simulink model "case1"  (R2024b)
settings: Solver=FixedStepAuto  StartTime=0  StopTime=1  FixedStep=1e-7  RelTol=1e-3
values from neighbouring files (symbols this model uses):
  SG_D_1_D = 0.01056    [IEEE9_case_parameters.m]    (also in case1_parameters.m; case2_parameters.m; case3_parameters.m; case4_parameters.m)
  SG_D_1_EnableSaturation = 0    [IEEE9_case_parameters.m]    (also in case1_parameters.m; case2_parameters.m; case3_parameters.m; case4_parameters.m)
  SG_D_1_f0 = 60    [IEEE9_case_parameters.m]    (also in case1_parameters.m; case2_parameters.m; case3_parameters.m; case4_parameters.m)
  SG_D_1_H = 7.5    [IEEE9_case_parameters.m]    (also in case1_parameters.m; case2_parameters.m; case3_parameters.m; case4_parameters.m)
  SG_D_1_K_A = 20    [IEEE9_case_parameters.m]    (also in case1_parameters.m; case2_parameters.m; case3_parameters.m; case4_parameters.m)
  SG_D_1_K_E = 1.000000e+1    (= 10)    [IEEE9_case_parameters.m]    (also in case1_parameters.m; case2_parameters.m; case3_parameters.m; case4_parameters.m)
  SG_D_1_K_F = 2.363    [IEEE9_case_parameters.m]    (also in case1_parameters.m; case2_parameters.m; case3_parameters.m; case4_parameters.m)
  SG_D_1_K_s = 0.5    [IEEE9_case_parameters.m]    (also in case1_parameters.m = 5; case2_parameters.m = 5; case3_parameters.m = 5; case4_parameters.m = 5)
  SG_D_1_R_a = 0.001088    [IEEE9_case_parameters.m]    (also in case1_parameters.m; case2_parameters.m; case3_parameters.m; case4_parameters.m)
  SG_D_1_S_A = 1    [IEEE9_case_parameters.m]    (also in case1_parameters.m; case2_parameters.m; case3_parameters.m; case4_parameters.m)
  SG_D_1_S_B = 0.103    [IEEE9_case_parameters.m]    (also in case1_parameters.m; case2_parameters.m; case3_parameters.m; case4_parameters.m)
  SG_D_1_S_N = 10.659857    [IEEE9_case_parameters.m]    (also in case1_parameters.m; case2_parameters.m; case3_parameters.m; case4_parameters.m)
  SG_D_1_SpeedPara = 200    [IEEE9_case_parameters.m]    (also in case1_parameters.m; case2_parameters.m; case3_parameters.m; case4_parameters.m)
  SG_D_1_T_0 = 0.720173    [IEEE9_case_parameters.m]    (also in case1_parameters.m = 0.755522; case2_parameters.m = 0.808931; case3_parameters.m = 0.869402; case4_parameters.m = 0.729316)
  SG_D_1_T_1 = 0.3    [IEEE9_case_parameters.m]    (also in case1_parameters.m; case2_parameters.m; case3_parameters.m; case4_parameters.m)
  SG_D_1_T_2 = 0.05    [IEEE9_case_parameters.m]    (also in case1_parameters.m; case2_parameters.m; case3_parameters.m; case4_parameters.m)
  SG_D_1_T_3 = 0.02    [IEEE9_case_parameters.m]    (also in case1_parameters.m; case2_parameters.m; case3_parameters.m; case4_parameters.m)
  SG_D_1_T_4 = 0.005    [IEEE9_case_parameters.m]    (also in case1_parameters.m; case2_parameters.m; case3_parameters.m; case4_parameters.m)
  SG_D_1_T_A = 0.02    [IEEE9_case_parameters.m]    (also in case1_parameters.m; case2_parameters.m; case3_parameters.m; case4_parameters.m)
  SG_D_1_T_dd = 8.000000e+0    (= 8)    [IEEE9_case_parameters.m]    (also in case1_parameters.m; case2_parameters.m; case3_parameters.m; case4_parameters.m)
  SG_D_1_T_ddd = 0.04    [IEEE9_case_parameters.m]    (also in case1_parameters.m; case2_parameters.m; case3_parameters.m; case4_parameters.m)
  SG_D_1_T_E = 0.314    [IEEE9_case_parameters.m]    (also in case1_parameters.m; case2_parameters.m; case3_parameters.m; case4_parameters.m)
  SG_D_1_T_F = 0.35    [IEEE9_case_parameters.m]    (also in case1_parameters.m; case2_parameters.m; case3_parameters.m; case4_parameters.m)
  SG_D_1_T_qd = 0.8    [IEEE9_case_parameters.m]    (also in case1_parameters.m; case2_parameters.m; case3_parameters.m; case4_parameters.m)
  SG_D_1_T_qdd = 0.02    [IEEE9_case_parameters.m]    (also in case1_parameters.m; case2_parameters.m; case3_parameters.m; case4_parameters.m)
  SG_D_1_T_speed = 0.1    [IEEE9_case_parameters.m]    (also in case1_parameters.m = 200; case2_parameters.m = 200; case3_parameters.m = 200; case4_parameters.m = 200)
  SG_D_1_T_w = 0.5    [IEEE9_case_parameters.m]    (also in case1_parameters.m; case2_parameters.m; case3_parameters.m; case4_parameters.m)
  SG_D_1_V_ref = 1.990276    [IEEE9_case_parameters.m]    (also in case1_parameters.m = 2.042296; case2_parameters.m = 2.051388; case3_parameters.m = 2.089584; case4_parameters.m = 2.01845)
  SG_D_1_w_ref = 376.991118    [IEEE9_case_parameters.m]    (also in case1_parameters.m; case2_parameters.m; case3_parameters.m; case4_parameters.m)
  SG_D_1_wb = 6.000000e+1    (= 60)    [IEEE9_case_parameters.m]    (also in case1_parameters.m; case2_parameters.m; case3_parameters.m; case4_parameters.m)
  SG_D_1_x_d = 1.9    [IEEE9_case_parameters.m]    (also in case1_parameters.m; case2_parameters.m; case3_parameters.m; case4_parameters.m)
  SG_D_1_x_dd = 0.302    [IEEE9_case_parameters.m]    (also in case1_parameters.m; case2_parameters.m; case3_parameters.m; case4_parameters.m)
  SG_D_1_x_ddd = 0.204    [IEEE9_case_parameters.m]    (also in case1_parameters.m; case2_parameters.m; case3_parameters.m; case4_parameters.m)
  SG_D_1_x_l = 0.05    [IEEE9_case_parameters.m]    (also in case1_parameters.m; case2_parameters.m; case3_parameters.m; case4_parameters.m)
  SG_D_1_x_q = 1.3    [IEEE9_case_parameters.m]    (also in case1_parameters.m; case2_parameters.m; case3_parameters.m; case4_parameters.m)
  SG_D_1_x_qd = 0.5    [IEEE9_case_parameters.m]    (also in case1_parameters.m; case2_parameters.m; case3_parameters.m; case4_parameters.m)
  SG_D_1_x_qdd = 0.3    [IEEE9_case_parameters.m]    (also in case1_parameters.m; case2_parameters.m; case3_parameters.m; case4_parameters.m)
  SG_D_2_D = 0.02    [IEEE9_case_parameters.m]    (also in case1_parameters.m; case2_parameters.m; case3_parameters.m; case4_parameters.m)
  SG_D_2_EnableSaturation = 0    [IEEE9_case_parameters.m]    (also in case1_parameters.m; case2_parameters.m; case3_parameters.m; case4_parameters.m)
  SG_D_2_f0 = 60    [IEEE9_case_parameters.m]    (also in case1_parameters.m; case2_parameters.m; case3_parameters.m; case4_parameters.m)
  SG_D_2_H = 8.000000e+0    (= 8)    [IEEE9_case_parameters.m]    (also in case1_parameters.m; case2_parameters.m; case3_parameters.m; case4_parameters.m)
  SG_D_2_K_A = 20    [IEEE9_case_parameters.m]    (also in case1_parameters.m; case2_parameters.m; case3_parameters.m; case4_parameters.m)
  SG_D_2_K_E = 1.000000e+1    (= 10)    [IEEE9_case_parameters.m]    (also in case1_parameters.m; case2_parameters.m; case3_parameters.m; case4_parameters.m)
  SG_D_2_K_F = 2.363    [IEEE9_case_parameters.m]    (also in case1_parameters.m; case2_parameters.m; case3_parameters.m; case4_parameters.m)
  SG_D_2_K_s = 0.5    [IEEE9_case_parameters.m]    (also in case1_parameters.m = 4; case2_parameters.m = 4; case3_parameters.m = 4; case4_parameters.m = 4)
  SG_D_2_R_a = 0.001088    [IEEE9_case_parameters.m]    (also in case1_parameters.m; case2_parameters.m; case3_parameters.m; case4_parameters.m)
  SG_D_2_S_A = 1    [IEEE9_case_parameters.m]    (also in case1_parameters.m; case2_parameters.m; case3_parameters.m; case4_parameters.m)
  SG_D_2_S_B = 0.103    [IEEE9_case_parameters.m]    (also in case1_parameters.m; case2_parameters.m; case3_parameters.m; case4_parameters.m)
  SG_D_2_S_N = 10.659857    [IEEE9_case_parameters.m]    (also in case1_parameters.m; case2_parameters.m; case3_parameters.m; case4_parameters.m)
  SG_D_2_SpeedPara = 200    [IEEE9_case_parameters.m]    (also in case1_parameters.m; case2_parameters.m; case3_parameters.m; case4_parameters.m)
  SG_D_2_T_0 = 1.632913    [IEEE9_case_parameters.m]    (also in case1_parameters.m = 1.632925; case2_parameters.m = 1.632915; case3_parameters.m = 1.632914; case4_parameters.m = 1.632927)
  SG_D_2_T_1 = 0.2    [IEEE9_case_parameters.m]    (also in case1_parameters.m; case2_parameters.m; case3_parameters.m; case4_parameters.m)
  SG_D_2_T_2 = 0.05    [IEEE9_case_parameters.m]    (also in case1_parameters.m; case2_parameters.m; case3_parameters.m; case4_parameters.m)
  SG_D_2_T_3 = 0.02    [IEEE9_case_parameters.m]    (also in case1_parameters.m; case2_parameters.m; case3_parameters.m; case4_parameters.m)
  SG_D_2_T_4 = 0.005    [IEEE9_case_parameters.m]    (also in case1_parameters.m; case2_parameters.m; case3_parameters.m; case4_parameters.m)
  SG_D_2_T_A = 0.02    [IEEE9_case_parameters.m]    (also in case1_parameters.m; case2_parameters.m; case3_parameters.m; case4_parameters.m)
  SG_D_2_T_dd = 7.9    [IEEE9_case_parameters.m]    (also in case1_parameters.m; case2_parameters.m; case3_parameters.m; case4_parameters.m)
  SG_D_2_T_ddd = 0.04    [IEEE9_case_parameters.m]    (also in case1_parameters.m; case2_parameters.m; case3_parameters.m; case4_parameters.m)
  SG_D_2_T_E = 0.314    [IEEE9_case_parameters.m]    (also in case1_parameters.m; case2_parameters.m; case3_parameters.m; case4_parameters.m)
  SG_D_2_T_F = 0.35    [IEEE9_case_parameters.m]    (also in case1_parameters.m; case2_parameters.m; case3_parameters.m; case4_parameters.m)
  SG_D_2_T_qd = 0.8    [IEEE9_case_parameters.m]    (also in case1_parameters.m; case2_parameters.m; case3_parameters.m; case4_parameters.m)
  SG_D_2_T_qdd = 0.015    [IEEE9_case_parameters.m]    (also in case1_parameters.m; case2_parameters.m; case3_parameters.m; case4_parameters.m)
  SG_D_2_T_speed = 0.1    [IEEE9_case_parameters.m]    (also in case1_parameters.m = 150; case2_parameters.m = 150; case3_parameters.m = 150; case4_parameters.m = 150)
  SG_D_2_T_w = 0.35    [IEEE9_case_parameters.m]    (also in case1_parameters.m; case2_parameters.m; case3_parameters.m; case4_parameters.m)
  SG_D_2_V_ref = 2.58547    [IEEE9_case_parameters.m]    (also in case1_parameters.m = 2.597896; case2_parameters.m = 2.587136; case3_parameters.m = 2.586042; case4_parameters.m = 2.599679)
  SG_D_2_w_ref = 376.991118    [IEEE9_case_parameters.m]    (also in case1_parameters.m; case2_parameters.m; case3_parameters.m; case4_parameters.m)
  SG_D_2_wb = 6.000000e+1    (= 60)    [IEEE9_case_parameters.m]    (also in case1_parameters.m; case2_parameters.m; case3_parameters.m; case4_parameters.m)
  SG_D_2_x_d = 1.8    [IEEE9_case_parameters.m]    (also in case1_parameters.m; case2_parameters.m; case3_parameters.m; case4_parameters.m)
  SG_D_2_x_dd = 0.302    [IEEE9_case_parameters.m]    (also in case1_parameters.m; case2_parameters.m; case3_parameters.m; case4_parameters.m)
  SG_D_2_x_ddd = 0.204    [IEEE9_case_parameters.m]    (also in case1_parameters.m; case2_parameters.m; case3_parameters.m; case4_parameters.m)
  SG_D_2_x_l = 0.05    [IEEE9_case_parameters.m]    (also in case1_parameters.m; case2_parameters.m; case3_parameters.m; case4_parameters.m)
  SG_D_2_x_q = 1.25    [IEEE9_case_parameters.m]    (also in case1_parameters.m; case2_parameters.m; case3_parameters.m; case4_parameters.m)
  SG_D_2_x_qd = 0.5    [IEEE9_case_parameters.m]    (also in case1_parameters.m; case2_parameters.m; case3_parameters.m; case4_parameters.m)
  SG_D_2_x_qdd = 0.3    [IEEE9_case_parameters.m]    (also in case1_parameters.m; case2_parameters.m; case3_parameters.m; case4_parameters.m)
  SG_D_3_D = 0.02    [IEEE9_case_parameters.m]    (also in case1_parameters.m; case2_parameters.m; case3_parameters.m; case4_parameters.m)
  SG_D_3_EnableSaturation = 0    [IEEE9_case_parameters.m]    (also in case1_parameters.m; case2_parameters.m; case3_parameters.m; case4_parameters.m)
  SG_D_3_f0 = 60    [IEEE9_case_parameters.m]    (also in case1_parameters.m; case2_parameters.m; case3_parameters.m; case4_parameters.m)
  SG_D_3_H = 7.7    [IEEE9_case_parameters.m]    (also in case1_parameters.m; case2_parameters.m; case3_parameters.m; case4_parameters.m)
  SG_D_3_K_A = 20    [IEEE9_case_parameters.m]    (also in case1_parameters.m; case2_parameters.m; case3_parameters.m; case4_parameters.m)
  SG_D_3_K_E = 1.000000e+1    (= 10)    [IEEE9_case_parameters.m]    (also in case1_parameters.m; case2_parameters.m; case3_parameters.m; case4_parameters.m)
  SG_D_3_K_F = 2.363    [IEEE9_case_parameters.m]    (also in case1_parameters.m; case2_parameters.m; case3_parameters.m; case4_parameters.m)
  SG_D_3_K_s = 0.2    [IEEE9_case_parameters.m]    (also in case1_parameters.m = 2; case2_parameters.m = 2; case3_parameters.m = 2; case4_parameters.m = 2)
  SG_D_3_R_a = 0.001088    [IEEE9_case_parameters.m]    (also in case1_parameters.m; case2_parameters.m; case3_parameters.m; case4_parameters.m)
  SG_D_3_S_A = 1    [IEEE9_case_parameters.m]    (also in case1_parameters.m; case2_parameters.m; case3_parameters.m; case4_parameters.m)
  SG_D_3_S_B = 0.103    [IEEE9_case_parameters.m]    (also in case1_parameters.m; case2_parameters.m; case3_parameters.m; case4_parameters.m)
  SG_D_3_S_N = 10.659857    [IEEE9_case_parameters.m]    (also in case1_parameters.m; case2_parameters.m; case3_parameters.m; case4_parameters.m)
  SG_D_3_SpeedPara = 200    [IEEE9_case_parameters.m]    (also in case1_parameters.m; case2_parameters.m; case3_parameters.m; case4_parameters.m)
  SG_D_3_T_0 = 0.850788    [IEEE9_case_parameters.m]    (also in case1_parameters.m = 0.850786; case2_parameters.m = 0.850787; case3_parameters.m; case4_parameters.m = 0.850786)
  SG_D_3_T_1 = 0.2    [IEEE9_case_parameters.m]    (also in case1_parameters.m; case2_parameters.m; case3_parameters.m; case4_parameters.m)
  SG_D_3_T_2 = 0.05    [IEEE9_case_parameters.m]    (also in case1_parameters.m; case2_parameters.m; case3_parameters.m; case4_parameters.m)
  SG_D_3_T_3 = 0.02    [IEEE9_case_parameters.m]    (also in case1_parameters.m; case2_parameters.m; case3_parameters.m; case4_parameters.m)
  SG_D_3_T_4 = 0.005    [IEEE9_case_parameters.m]    (also in case1_parameters.m; case2_parameters.m; case3_parameters.m; case4_parameters.m)
  SG_D_3_T_A = 0.02    [IEEE9_case_parameters.m]    (also in case1_parameters.m; case2_parameters.m; case3_parameters.m; case4_parameters.m)
  SG_D_3_T_dd = 8.1    [IEEE9_case_parameters.m]    (also in case1_parameters.m; case2_parameters.m; case3_parameters.m; case4_parameters.m)
  SG_D_3_T_ddd = 0.04    [IEEE9_case_parameters.m]    (also in case1_parameters.m; case2_parameters.m; case3_parameters.m; case4_parameters.m)
  SG_D_3_T_E = 0.314    [IEEE9_case_parameters.m]    (also in case1_parameters.m; case2_parameters.m; case3_parameters.m; case4_parameters.m)
  SG_D_3_T_F = 0.35    [IEEE9_case_parameters.m]    (also in case1_parameters.m; case2_parameters.m; case3_parameters.m; case4_parameters.m)
  SG_D_3_T_qd = 0.8    [IEEE9_case_parameters.m]    (also in case1_parameters.m; case2_parameters.m; case3_parameters.m; case4_parameters.m)
  SG_D_3_T_qdd = 0.015    [IEEE9_case_parameters.m]    (also in case1_parameters.m; case2_parameters.m; case3_parameters.m; case4_parameters.m)
  SG_D_3_T_speed = 0.1    [IEEE9_case_parameters.m]    (also in case1_parameters.m = 180; case2_parameters.m = 180; case3_parameters.m = 180; case4_parameters.m = 180)
  SG_D_3_T_w = 0.4    [IEEE9_case_parameters.m]    (also in case1_parameters.m; case2_parameters.m; case3_parameters.m; case4_parameters.m)
  SG_D_3_V_ref = 1.892727    [IEEE9_case_parameters.m]    (also in case1_parameters.m = 1.906439; case2_parameters.m = 1.895535; case3_parameters.m = 1.892105; case4_parameters.m = 1.906598)
  SG_D_3_w_ref = 376.991118    [IEEE9_case_parameters.m]    (also in case1_parameters.m; case2_parameters.m; case3_parameters.m; case4_parameters.m)
  SG_D_3_wb = 6.000000e+1    (= 60)    [IEEE9_case_parameters.m]    (also in case1_parameters.m; case2_parameters.m; case3_parameters.m; case4_parameters.m)
  SG_D_3_x_d = 1.85    [IEEE9_case_parameters.m]    (also in case1_parameters.m; case2_parameters.m; case3_parameters.m; case4_parameters.m)
  SG_D_3_x_dd = 0.302    [IEEE9_case_parameters.m]    (also in case1_parameters.m; case2_parameters.m; case3_parameters.m; case4_parameters.m)
  SG_D_3_x_ddd = 0.204    [IEEE9_case_parameters.m]    (also in case1_parameters.m; case2_parameters.m; case3_parameters.m; case4_parameters.m)
  SG_D_3_x_l = 0.05    [IEEE9_case_parameters.m]    (also in case1_parameters.m; case2_parameters.m; case3_parameters.m; case4_parameters.m)
  SG_D_3_x_q = 1.2    [IEEE9_case_parameters.m]    (also in case1_parameters.m; case2_parameters.m; case3_parameters.m; case4_parameters.m)
  SG_D_3_x_qd = 0.5    [IEEE9_case_parameters.m]    (also in case1_parameters.m; case2_parameters.m; case3_parameters.m; case4_parameters.m)
  SG_D_3_x_qdd = 0.3    [IEEE9_case_parameters.m]    (also in case1_parameters.m; case2_parameters.m; case3_parameters.m; case4_parameters.m)
(part 7 of 12)

== system case1/SG_D_2/T_e_SG_D_2_block ==
  note: T_e_SG_D_2 in case1
      | $-\frac{\psi _{d,\mathrm{SG},D,2}\,\left(\psi _{q,\mathrm{SG},D,2}+\frac{\psi _{\mathrm{gq},\mathrm{SG},D,2}\,\left(x_{l}-x_{\mathrm{qdd}}\right)}{x_{l}-x_{\mathrm{qd}}}+\frac{\psi _{\mathrm{kq},\mathrm{SG},D,2}\,\left(x_{\mathrm{qd}}-x_{\mathrm{qdd}}\right)}{x_{l}-x_{\mathrm{qd}}}\right)}{x_{\mathrm{qdd}}}-\frac{\psi _{q,\mathrm{SG},D,2}\,\left(\frac{\psi _{\mathrm{1d},\mathrm{SG},D,2}\,\left(x_{\mathrm{dd}}-x_{\mathrm{ddd}}\right)}{x_{\mathrm{dd}}-x_{l}}-\psi _{d,\mathrm{SG},D,2}+\frac{\psi _{\mathrm{fd},\mathrm{SG},D,2}\,\left(x_{\mathrm{ddd}}-x_{l}\right)}{x_{\mathrm{dd}}-x_{l}}\right)}{x_{\mathrm{ddd}}}$
      | Automatically generated on 2025-10-31 18:49:09 .
  State_psi_d_SG_D_2_d17d7 : Inport
  State_psi_gq_SG_D_2_50ede : Inport  Port=2
  State_psi_kq_SG_D_2_ad282 : Inport  Port=3
  State_psi_q_SG_D_2_25b32 : Inport  Port=4
  State_psi_q_SG_D_2_fddea : Inport  Port=5
  State_psi_1d_SG_D_2_6821c : Inport  Port=6
  State_psi_d_SG_D_2_3bce2 : Inport  Port=7
  State_psi_fd_SG_D_2_27f6e : Inport  Port=8
  Add_23b6a : Sum
  Add_42760 : Sum
  Add_98a11 : Sum
  Add_aa7f3 : Sum
  Add_c8d0f : Sum
  Add_d49e1 : Sum
  Constant_-1_0fe01 : Constant  Value=-1
  Constant_-1_35857 : Constant  Value=-1
  Constant_-1_5d818 : Constant  Value=-1
  Constant_-1_78a66 : Constant  Value=-1
  Constant_-1_c3573 : Constant  Value=-1
  Constant_x_dd_09cbb : Constant  Value=x_dd
  Constant_x_dd_48c2b : Constant  Value=x_dd
  Constant_x_dd_a60eb : Constant  Value=x_dd
  Constant_x_ddd_2410b : Constant  Value=x_ddd
  Constant_x_ddd_26014 : Constant  Value=x_ddd
  Constant_x_ddd_6425f : Constant  Value=x_ddd
  Constant_x_l_05096 : Constant  Value=x_l
  Constant_x_l_3e3b1 : Constant  Value=x_l
  Constant_x_l_8c6a1 : Constant  Value=x_l
  Constant_x_l_93e72 : Constant  Value=x_l
  Constant_x_l_aba57 : Constant  Value=x_l
  Constant_x_l_c3be9 : Constant  Value=x_l
  Constant_x_qd_320b4 : Constant  Value=x_qd
  Constant_x_qd_56ce7 : Constant  Value=x_qd
  Constant_x_qd_8b2ca : Constant  Value=x_qd
  Constant_x_qdd_735f7 : Constant  Value=x_qdd
  Constant_x_qdd_e2b73 : Constant  Value=x_qdd
  Constant_x_qdd_e8dda : Constant  Value=x_qdd
  Divide_3759f : Product  Inputs=*/
  Divide_3be13 : Product  Inputs=*/
  Divide_9f252 : Product  Inputs=*/
  Divide_a3918 : Product  Inputs=*/
  Divide_aa95e : Product  Inputs=*/
  Divide_b0829 : Product  Inputs=*/
  Product_024a1 : Product
  Product_03878 : Product
  Product_2d239 : Product
  Product_3b454 : Product
  Product_4d8bd : Product
  Product_50cc2 : Product
  Product_5812c : Product
  Product_63870 : Product
  Product_da8e1 : Product
  Product_df83d : Product
  Product_e3721 : Product
  Subtract_283ed : Sum  Inputs=+-
  Subtract_3343d : Sum  Inputs=+-
  Subtract_51917 : Sum  Inputs=+-
  Subtract_708f3 : Sum  Inputs=+-
  Subtract_77632 : Sum  Inputs=+-
  Subtract_c6d03 : Sum  Inputs=+-
  Subtract_eb7e9 : Sum  Inputs=+-
  Blockout_T_e_SG_D_2_b65d9 : Outport
  wires:
  Constant_-1_5d818/1 -> Product_df83d/1
  Divide_a3918/1 -> Subtract_eb7e9/1
  Constant_-1_35857/1 -> Product_50cc2/1
  Constant_x_l_8c6a1/1 -> Product_50cc2/2
  Constant_x_qd_320b4/1 -> Subtract_51917/1
  Product_024a1/1 -> Divide_a3918/1
  Product_50cc2/1 -> Add_c8d0f/1
  Divide_aa95e/1 -> Subtract_3343d/2
  Constant_x_qdd_735f7/1 -> Subtract_51917/2
  Constant_x_qdd_e8dda/1 -> Divide_b0829/2
  Constant_x_ddd_6425f/1 -> Subtract_77632/2
  Constant_x_qdd_e2b73/1 -> Add_c8d0f/2
  Constant_x_l_93e72/1 -> Product_df83d/2
  Constant_-1_0fe01/1 -> Product_e3721/1
  Constant_x_l_3e3b1/1 -> Product_e3721/2
  Constant_-1_78a66/1 -> Product_03878/1
  State_psi_1d_SG_D_2_6821c/1 -> Product_03878/2
  Constant_x_dd_09cbb/1 -> Subtract_77632/1
  Divide_3be13/1 -> Subtract_eb7e9/2
  State_psi_gq_SG_D_2_50ede/1 -> Product_024a1/1
  Add_c8d0f/1 -> Product_024a1/2
  Subtract_eb7e9/1 -> Add_d49e1/1
  Constant_x_dd_48c2b/1 -> Subtract_708f3/1
  Product_df83d/1 -> Add_98a11/1
  Product_4d8bd/1 -> Product_5812c/1
  Constant_x_qd_56ce7/1 -> Add_98a11/2
  State_psi_kq_SG_D_2_ad282/1 -> Product_da8e1/1
  Subtract_51917/1 -> Product_da8e1/2
  Product_e3721/1 -> Add_aa7f3/1
  State_psi_q_SG_D_2_fddea/1 -> Product_63870/1
  Constant_x_qd_8b2ca/1 -> Add_aa7f3/2
  Product_03878/1 -> Product_2d239/1
  Divide_3759f/1 -> Add_23b6a/2
  Subtract_77632/1 -> Product_2d239/2
  Constant_x_l_c3be9/1 -> Subtract_708f3/2
  Constant_x_ddd_26014/1 -> Subtract_c6d03/1
  Constant_x_dd_a60eb/1 -> Subtract_283ed/1
  Constant_x_l_05096/1 -> Subtract_c6d03/2
  Add_23b6a/1 -> Blockout_T_e_SG_D_2_b65d9/1
  Add_98a11/1 -> Divide_a3918/2
  Product_da8e1/1 -> Divide_3be13/1
  Product_5812c/1 -> Divide_b0829/1
  State_psi_d_SG_D_2_d17d7/1 -> Product_4d8bd/2
  Add_aa7f3/1 -> Divide_3be13/2
  Product_2d239/1 -> Divide_9f252/1
  Subtract_708f3/1 -> Divide_9f252/2
  Constant_x_l_aba57/1 -> Subtract_283ed/2
  State_psi_fd_SG_D_2_27f6e/1 -> Product_3b454/1
  Constant_x_ddd_2410b/1 -> Divide_3759f/2
  Product_63870/1 -> Divide_3759f/1
  Subtract_c6d03/1 -> Product_3b454/2
  Divide_9f252/1 -> Add_42760/1
  State_psi_d_SG_D_2_3bce2/1 -> Add_42760/2
  Add_42760/1 -> Subtract_3343d/1
  Product_3b454/1 -> Divide_aa95e/1
  Subtract_283ed/1 -> Divide_aa95e/2
  Constant_-1_c3573/1 -> Product_4d8bd/1
  State_psi_q_SG_D_2_25b32/1 -> Add_d49e1/2
  Add_d49e1/1 -> Product_5812c/2
  Subtract_3343d/1 -> Product_63870/2
  Divide_b0829/1 -> Add_23b6a/1

== system case1/SG_D_2/d_E_fd_SG_D_2_block ==
  note: d_E_fd_SG_D_2 in case1
      | $\frac{V_{f,\mathrm{SG},D,2}-E_{\mathrm{fd},\mathrm{SG},D,2}\,K_{E}}{T_{E}}$
      | Automatically generated on 2025-10-31 18:48:51 .
  State_E_fd_SG_D_2_f3b44 : Inport
  State_V_f_SG_D_2_853e9 : Inport  Port=2
  Add_3a545 : Sum
  Constant_-1_cf921 : Constant  Value=-1
  Constant_K_E_ca9b5 : Constant  Value=K_E
  Constant_T_E_8d026 : Constant  Value=T_E
  Divide_8de38 : Product  Inputs=*/
  Product_ab2ba : Product
  Product_fb98c : Product
  Blockout_d_E_fd_SG_D_2_6e556 : Outport
  wires:
  Constant_-1_cf921/1 -> Product_fb98c/1
  State_E_fd_SG_D_2_f3b44/1 -> Product_fb98c/2
  Product_fb98c/1 -> Product_ab2ba/1
  Constant_K_E_ca9b5/1 -> Product_ab2ba/2
  Product_ab2ba/1 -> Add_3a545/1
  Constant_T_E_8d026/1 -> Divide_8de38/2
  State_V_f_SG_D_2_853e9/1 -> Add_3a545/2
  Add_3a545/1 -> Divide_8de38/1
  Divide_8de38/1 -> Blockout_d_E_fd_SG_D_2_6e556/1

== system case1/SG_D_2/d_Px_1_SG_D_2_block ==
  note: d_Px_1_SG_D_2 in case1
      | $\frac{w_{\mathrm{SG},D,2}-2\,\pi \,f_{0}}{T_{w}}-\frac{\mathrm{Px}_{1,\mathrm{SG},D,2}}{T_{w}}$
      | Automatically generated on 2025-10-31 18:48:52 .
  State_Px_1_SG_D_2_dab25 : Inport
  State_w_SG_D_2_a2171 : Inport  Port=2
  Add_2ab8a : Sum
  Add_360ba : Sum
  Constant_-1_2edce : Constant  Value=-1
  Constant_-2.0_2f753 : Constant  Value=-2.0
  Constant_T_w_0f960 : Constant  Value=T_w
  Constant_T_w_7a6f9 : Constant  Value=T_w
  Constant_f0_1a930 : Constant  Value=f0
  Constant_pi_2d2fd : Constant  Value=pi
  Divide_5c21f : Product  Inputs=*/
  Divide_d4372 : Product  Inputs=*/
  Product_0634f : Product
  Product_9fae9 : Product
  Product_e2389 : Product
  Blockout_d_Px_1_SG_D_2_8641a : Outport
  wires:
  Constant_-2.0_2f753/1 -> Product_e2389/1
  State_w_SG_D_2_a2171/1 -> Add_360ba/2
  Constant_pi_2d2fd/1 -> Product_e2389/2
  Product_e2389/1 -> Product_9fae9/1
  Constant_f0_1a930/1 -> Product_9fae9/2
  Constant_-1_2edce/1 -> Product_0634f/1
  State_Px_1_SG_D_2_dab25/1 -> Product_0634f/2
  Product_9fae9/1 -> Add_360ba/1
  Product_0634f/1 -> Divide_5c21f/1
  Constant_T_w_7a6f9/1 -> Divide_5c21f/2
  Add_360ba/1 -> Divide_d4372/1
  Constant_T_w_0f960/1 -> Divide_d4372/2
  Divide_5c21f/1 -> Add_2ab8a/1
  Divide_d4372/1 -> Add_2ab8a/2
  Add_2ab8a/1 -> Blockout_d_Px_1_SG_D_2_8641a/1

== system case1/SG_D_2/d_Px_2_SG_D_2_block ==
  note: d_Px_2_SG_D_2 in case1
      | $\frac{\mathrm{Px}_{1,\mathrm{SG},D,2}-T_{2}\,\left(\frac{\mathrm{Px}_{1,\mathrm{SG},D,2}}{T_{w}}-\frac{w_{\mathrm{SG},D,2}-2\,\pi \,f_{0}}{T_{w}}\right)}{T_{1}}-\frac{\mathrm{Px}_{2,\mathrm{SG},D,2}}{T_{1}}$
      | Automatically generated on 2025-10-31 18:48:54 .
  State_Px_2_SG_D_2_5b382 : Inport
  State_Px_1_SG_D_2_4a486 : Inport  Port=2
  State_Px_1_SG_D_2_0c9fb : Inport  Port=3
  State_w_SG_D_2_d1507 : Inport  Port=4
  Add_18b9e : Sum
  Add_3fe59 : Sum
  Add_c7352 : Sum
  Add_d49e9 : Sum
  Constant_-1_6f4d2 : Constant  Value=-1
  Constant_-1_c3157 : Constant  Value=-1
  Constant_-2.0_b9580 : Constant  Value=-2.0
  Constant_T_1_13a70 : Constant  Value=T_1
  Constant_T_1_ed9d4 : Constant  Value=T_1
  Constant_T_2_96a07 : Constant  Value=T_2
  Constant_T_w_418d3 : Constant  Value=T_w
  Constant_T_w_d1cac : Constant  Value=T_w
  Constant_f0_175ae : Constant  Value=f0
  Constant_pi_15b61 : Constant  Value=pi
  Divide_20c9a : Product  Inputs=*/
  Divide_226ff : Product  Inputs=*/
  Divide_b3086 : Product  Inputs=*/
  Divide_b4a77 : Product  Inputs=*/
  Product_2b6c0 : Product
  Product_3964c : Product
  Product_3ddf0 : Product
  Product_57ea1 : Product
  Product_b09de : Product
  Blockout_d_Px_2_SG_D_2_74daf : Outport
  wires:
  Constant_-1_6f4d2/1 -> Product_3964c/1
  Constant_-2.0_b9580/1 -> Product_57ea1/1
  Product_3ddf0/1 -> Add_3fe59/2
  State_w_SG_D_2_d1507/1 -> Add_d49e9/2
  Constant_pi_15b61/1 -> Product_57ea1/2
  Product_57ea1/1 -> Product_b09de/1
  State_Px_1_SG_D_2_0c9fb/1 -> Product_2b6c0/2
  Constant_f0_175ae/1 -> Product_b09de/2
  State_Px_2_SG_D_2_5b382/1 -> Product_3964c/2
  Constant_-1_c3157/1 -> Product_2b6c0/1
  Product_b09de/1 -> Add_d49e9/1
  Product_2b6c0/1 -> Divide_20c9a/1
  Constant_T_w_418d3/1 -> Divide_20c9a/2
  Add_d49e9/1 -> Divide_226ff/1
  Constant_T_w_d1cac/1 -> Divide_226ff/2
  Divide_20c9a/1 -> Add_c7352/1
  Divide_226ff/1 -> Add_c7352/2
  Constant_T_2_96a07/1 -> Product_3ddf0/1
  Add_c7352/1 -> Product_3ddf0/2
  State_Px_1_SG_D_2_4a486/1 -> Add_3fe59/1
  Product_3964c/1 -> Divide_b4a77/1
  Constant_T_1_ed9d4/1 -> Divide_b4a77/2
  Add_3fe59/1 -> Divide_b3086/1
  Constant_T_1_13a70/1 -> Divide_b3086/2
  Divide_b4a77/1 -> Add_18b9e/1
  Divide_b3086/1 -> Add_18b9e/2
  Add_18b9e/1 -> Blockout_d_Px_2_SG_D_2_74daf/1

== system case1/SG_D_2/d_Px_3_SG_D_2_block ==
  note: d_Px_3_SG_D_2 in case1
      | $\frac{\mathrm{Px}_{2,\mathrm{SG},D,2}+T_{4}\,\left(\frac{\mathrm{Px}_{1,\mathrm{SG},D,2}-T_{2}\,\left(\frac{\mathrm{Px}_{1,\mathrm{SG},D,2}}{T_{w}}-\frac{w_{\mathrm{SG},D,2}-2\,\pi \,f_{0}}{T_{w}}\right)}{T_{1}}-\frac{\mathrm{Px}_{2,\mathrm{SG},D,2}}{T_{1}}\right)}{T_{3}}-\frac{\mathrm{Px}_{3,\mathrm{SG},D,2}}{T_{3}}$
      | Automatically generated on 2025-10-31 18:48:56 .
  State_Px_3_SG_D_2_47d77 : Inport
  State_Px_2_SG_D_2_29f59 : Inport  Port=2
  State_Px_2_SG_D_2_7bb9c : Inport  Port=3
  State_Px_1_SG_D_2_19b2b : Inport  Port=4
  State_Px_1_SG_D_2_dcab9 : Inport  Port=5
  State_w_SG_D_2_a0c55 : Inport  Port=6
  Add_3d0e3 : Sum
  Add_47d79 : Sum
  Add_6d748 : Sum
  Add_87dfc : Sum
  Add_ee9d2 : Sum
  Add_f6e5b : Sum
  Constant_-1_108d3 : Constant  Value=-1
  Constant_-1_5324d : Constant  Value=-1
  Constant_-1_e198b : Constant  Value=-1
  Constant_-2.0_fa96a : Constant  Value=-2.0
  Constant_T_1_54dee : Constant  Value=T_1
  Constant_T_1_77268 : Constant  Value=T_1
  Constant_T_2_4ef3a : Constant  Value=T_2
  Constant_T_3_2d523 : Constant  Value=T_3
  Constant_T_3_65e0e : Constant  Value=T_3
  Constant_T_4_eecbc : Constant  Value=T_4
  Constant_T_w_06642 : Constant  Value=T_w
  Constant_T_w_ebade : Constant  Value=T_w
  Constant_f0_84ceb : Constant  Value=f0
  Constant_pi_13dd1 : Constant  Value=pi
  Divide_29f72 : Product  Inputs=*/
  Divide_5d5f4 : Product  Inputs=*/
  Divide_88fe4 : Product  Inputs=*/
  Divide_b1524 : Product  Inputs=*/
  Divide_b4c03 : Product  Inputs=*/
  Divide_e48cb : Product  Inputs=*/
  Product_3cdd8 : Product
  Product_bc7a2 : Product
  Product_d2db5 : Product
  Product_d9325 : Product
  Product_e462f : Product
  Product_f4dd0 : Product
  Product_febdf : Product
  Blockout_d_Px_3_SG_D_2_3521b : Outport
  wires:
  Constant_-2.0_fa96a/1 -> Product_e462f/1
  State_w_SG_D_2_a0c55/1 -> Add_47d79/2
  Add_87dfc/1 -> Divide_88fe4/1
  Constant_pi_13dd1/1 -> Product_e462f/2
  Constant_-1_5324d/1 -> Product_d2db5/1
  Product_e462f/1 -> Product_d9325/1
  State_Px_2_SG_D_2_7bb9c/1 -> Product_d2db5/2
  State_Px_1_SG_D_2_dcab9/1 -> Product_f4dd0/2
  Divide_88fe4/1 -> Add_6d748/2
  Constant_f0_84ceb/1 -> Product_d9325/2
  Constant_-1_e198b/1 -> Product_f4dd0/1
  Product_d9325/1 -> Add_47d79/1
  Product_f4dd0/1 -> Divide_5d5f4/1
  Constant_T_w_06642/1 -> Divide_5d5f4/2
  Divide_e48cb/1 -> Add_6d748/1
  Add_47d79/1 -> Divide_b1524/1
  Product_3cdd8/1 -> Add_ee9d2/2
  Constant_T_w_ebade/1 -> Divide_b1524/2
  Divide_5d5f4/1 -> Add_f6e5b/1
  State_Px_1_SG_D_2_19b2b/1 -> Add_ee9d2/1
  Divide_b1524/1 -> Add_f6e5b/2
  Constant_-1_108d3/1 -> Product_febdf/1
  Constant_T_2_4ef3a/1 -> Product_3cdd8/1
  Add_f6e5b/1 -> Product_3cdd8/2
  Product_d2db5/1 -> Divide_b4c03/1
  Constant_T_1_77268/1 -> Divide_b4c03/2
  Add_ee9d2/1 -> Divide_29f72/1
  Constant_T_1_54dee/1 -> Divide_29f72/2
  Divide_b4c03/1 -> Add_3d0e3/1
  Divide_29f72/1 -> Add_3d0e3/2
  Constant_T_4_eecbc/1 -> Product_bc7a2/1
  Add_3d0e3/1 -> Product_bc7a2/2
  State_Px_3_SG_D_2_47d77/1 -> Product_febdf/2
  State_Px_2_SG_D_2_29f59/1 -> Add_87dfc/1
  Product_bc7a2/1 -> Add_87dfc/2
  Product_febdf/1 -> Divide_e48cb/1
  Constant_T_3_65e0e/1 -> Divide_e48cb/2
  Constant_T_3_2d523/1 -> Divide_88fe4/2
  Add_6d748/1 -> Blockout_d_Px_3_SG_D_2_3521b/1

== system case1/SG_D_2/d_R_f_SG_D_2_block ==
  note: d_R_f_SG_D_2 in case1
      | $-\frac{R_{f,\mathrm{SG},D,2}-\frac{E_{\mathrm{fd},\mathrm{SG},D,2}\,K_{F}}{T_{F}}}{T_{F}}$
      | Automatically generated on 2025-10-31 18:48:50 .
  State_E_fd_SG_D_2_b3245 : Inport
  State_R_f_SG_D_2_6bf16 : Inport  Port=2
  Constant_K_F_7db1c : Constant  Value=K_F
  Constant_T_F_34450 : Constant  Value=T_F
  Constant_T_F_ebc1c : Constant  Value=T_F
  Divide_5214b : Product  Inputs=*/
  Divide_b7c6b : Product  Inputs=*/
  Product_1adbd : Product
  Subtract_07eb8 : Sum  Inputs=+-
  Blockout_d_R_f_SG_D_2_3f1f3 : Outport
  wires:
  Constant_T_F_ebc1c/1 -> Divide_b7c6b/2
  State_E_fd_SG_D_2_b3245/1 -> Product_1adbd/1
  Constant_K_F_7db1c/1 -> Product_1adbd/2
  State_R_f_SG_D_2_6bf16/1 -> Subtract_07eb8/2
  Product_1adbd/1 -> Divide_b7c6b/1
  Divide_b7c6b/1 -> Subtract_07eb8/1
  Constant_T_F_34450/1 -> Divide_5214b/2
  Subtract_07eb8/1 -> Divide_5214b/1
  Divide_5214b/1 -> Blockout_d_R_f_SG_D_2_3f1f3/1

== system case1/SG_D_2/d_T_m_SG_D_2_block ==
  note: d_T_m_SG_D_2 in case1
      | $-\frac{T_{m,\mathrm{SG},D,2}-T_{0}+\frac{\mathrm{SpeedPara}\,\left(w_{\mathrm{SG},D,2}-w_{\mathrm{ref}}\right)}{2\,f_{0}\,\pi }}{T_{\mathrm{speed}}}$
      | Automatically generated on 2025-10-31 18:48:40 .
  State_w_SG_D_2_723fe : Inport
  State_T_m_SG_D_2_d95aa : Inport  Port=2
  Add_2d435 : Sum
  Add_4000c : Sum
  Constant_-1_6d274 : Constant  Value=-1
  Constant_2.0_e2dae : Constant  Value=2.0
  Constant_SpeedPara_e2c42 : Constant  Value=SpeedPara
  Constant_T_0_0cb7a : Constant  Value=T_0
  Constant_T_speed_2a494 : Constant  Value=T_speed
  Constant_f0_d8a90 : Constant  Value=f0
  Constant_pi_c99f1 : Constant  Value=pi
  Constant_w_ref_fc48a : Constant  Value=w_ref
  Divide_212f0 : Product  Inputs=*/
  Divide_b7dd9 : Product  Inputs=*/
  Product_2ae9f : Product
  Product_57384 : Product
  Product_9e400 : Product
  Product_e2475 : Product
  Subtract_2a667 : Sum  Inputs=+-
  Blockout_d_T_m_SG_D_2_43af5 : Outport
  wires:
  Constant_pi_c99f1/1 -> Product_e2475/2
  Constant_-1_6d274/1 -> Product_2ae9f/1
  Constant_w_ref_fc48a/1 -> Add_4000c/2
  State_w_SG_D_2_723fe/1 -> Product_2ae9f/2
  Product_2ae9f/1 -> Add_4000c/1
  Add_2d435/1 -> Subtract_2a667/1
  Add_4000c/1 -> Product_9e400/2
  Constant_2.0_e2dae/1 -> Product_e2475/1
  Constant_SpeedPara_e2c42/1 -> Product_9e400/1
  Product_e2475/1 -> Product_57384/1
  Constant_f0_d8a90/1 -> Product_57384/2
  Product_9e400/1 -> Divide_212f0/1
  Product_57384/1 -> Divide_212f0/2
  Divide_212f0/1 -> Add_2d435/1
  Constant_T_0_0cb7a/1 -> Add_2d435/2
  State_T_m_SG_D_2_d95aa/1 -> Subtract_2a667/2
  Subtract_2a667/1 -> Divide_b7dd9/1
  Constant_T_speed_2a494/1 -> Divide_b7dd9/2
  Divide_b7dd9/1 -> Blockout_d_T_m_SG_D_2_43af5/1

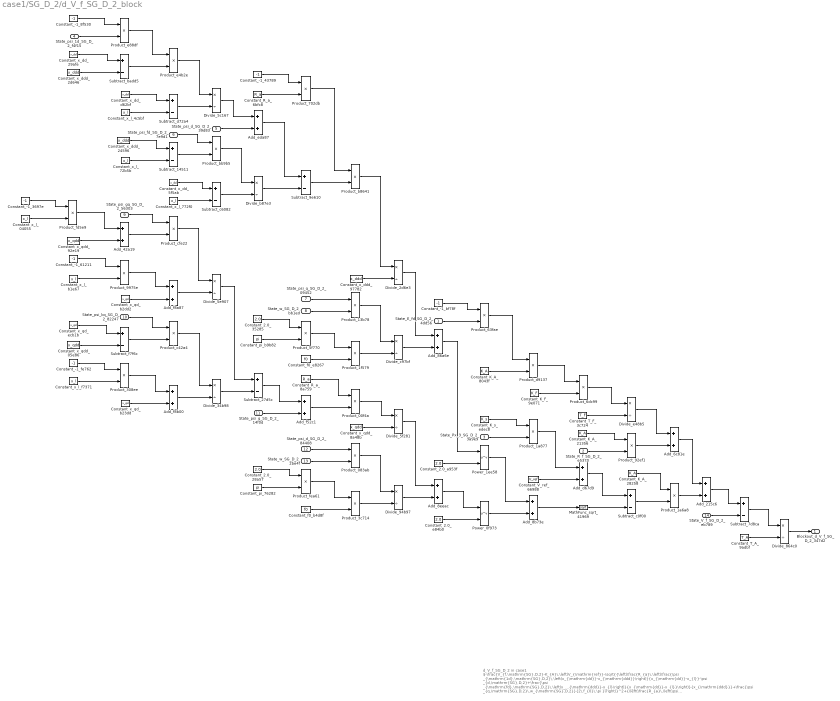
== system case1/SG_D_2/d_V_f_SG_D_2_block ==
  note: d_V_f_SG_D_2 in case1
      | $-\frac{V_{f,\mathrm{SG},D,2}-K_{A}\,\left(V_{\mathrm{ref}}-\sqrt{{\left(\frac{R_{a}\,\left(\frac{\psi _{\mathrm{1d},\mathrm{SG},D,2}\,\left(x_{\mathrm{dd}}-x_{\mathrm{ddd}}\right)}{x_{\mathrm{dd}}-x_{l}}-\psi _{d,\mathrm{SG},D,2}+\frac{\psi _{\mathrm{fd},\mathrm{SG},D,2}\,\left(x_{\mathrm{ddd}}-x_{l}\right)}{x_{\mathrm{dd}}-x_{l}}\right)}{x_{\mathrm{ddd}}}+\frac{\psi _{q,\mathrm{SG},D,2}\,w_{\mathrm{SG},D,2}}{2\,f_{0}\,\pi }\right)}^2+{\left(\frac{R_{a}\,\left(\psi _{q,\mathrm{SG},D,2}+\frac{\psi _{\mathrm{gq},\mathrm{SG},D,2}\,\left(x_{l}-x_{\mathrm{qdd}}\right)}{x_{l}-x_{\mathrm{qd}}}+\frac{\psi _{\mathrm{kq},\mathrm{SG},D,2}\,\left(x_{\mathrm{qd}}-x_{\mathrm{qdd}}\right)}{x_{l}-x_{\mathrm{qd}}}\right)}{x_{\mathrm{qdd}}}+\frac{\psi _{d,\mathrm{SG},D,2}\,w_{\mathrm{SG},D,2}}{2\,f_{0}\,\pi }\right)}^2}+K_{s}\,\mathrm{Px}_{3,\mathrm{SG},D,2}\right)-K_{A}\,R_{f,\mathrm{SG},D,2}+\frac{E_{\mathrm{fd},\mathrm{SG},D,2}\,K_{A}\,K_{F}}{T_{F}}}{T_{A}}$
      | Automatically generated on 2025-10-31 18:48:48 .
  State_E_fd_SG_D_2_4dd56 : Inport
  State_R_f_SG_D_2_e5370 : Inport  Port=2
  State_Px_3_SG_D_2_3a9e9 : Inport  Port=3
  State_psi_1d_SG_D_2_f4f15 : Inport  Port=4
  State_psi_d_SG_D_2_39d83 : Inport  Port=5
  State_psi_fd_SG_D_2_7e9d1 : Inport  Port=6
  State_psi_q_SG_D_2_09452 : Inport  Port=7
  State_w_SG_D_2_bb1ed : Inport  Port=8
  State_psi_gq_SG_D_2_56303 : Inport  Port=9
  State_psi_kq_SG_D_2_82247 : Inport  Port=10
  State_psi_q_SG_D_2_14f0d : Inport  Port=11
  State_psi_d_SG_D_2_84408 : Inport  Port=12
  State_w_SG_D_2_2be4f : Inport  Port=13
  State_V_f_SG_D_2_eb789 : Inport  Port=14
  Add_215c6 : Sum
  Add_42a19 : Sum
  Add_6c81e : Sum
  Add_86a6e : Sum
  Add_8b73e : Sum
  Add_8eeac : Sum
  Add_d67d9 : Sum
  Add_eda87 : Sum
  Add_f52c1 : Sum
  Add_f8a87 : Sum
  Add_f8b00 : Sum
  Constant_-1_3697e : Constant  Value=-1
  Constant_-1_43789 : Constant  Value=-1
  Constant_-1_61211 : Constant  Value=-1
  Constant_-1_8f530 : Constant  Value=-1
  Constant_-1_bf78f : Constant  Value=-1
  Constant_-1_fe762 : Constant  Value=-1
  Constant_2.0_28a57 : Constant  Value=2.0
  Constant_2.0_35285 : Constant  Value=2.0
  Constant_2.0_a953f : Constant  Value=2.0
  Constant_2.0_e84b0 : Constant  Value=2.0
  Constant_K_A_21356 : Constant  Value=K_A
  Constant_K_A_28258 : Constant  Value=K_A
  Constant_K_A_8043f : Constant  Value=K_A
  Constant_K_F_9e071 : Constant  Value=K_F
  Constant_K_s_edec8 : Constant  Value=K_s
  Constant_R_a_6bfc8 : Constant  Value=R_a
  Constant_R_a_8a759 : Constant  Value=R_a
  Constant_T_A_9adbf : Constant  Value=T_A
  Constant_T_F_3c724 : Constant  Value=T_F
  Constant_V_ref_66988 : Constant  Value=V_ref
  Constant_f0_b4d8f : Constant  Value=f0
  Constant_f0_e8267 : Constant  Value=f0
  Constant_pi_76282 : Constant  Value=pi
  Constant_pi_b9b82 : Constant  Value=pi
  Constant_x_dd_29afe : Constant  Value=x_dd
  Constant_x_dd_5f5ab : Constant  Value=x_dd
  Constant_x_dd_d62bf : Constant  Value=x_dd
  Constant_x_ddd_24596 : Constant  Value=x_ddd
  Constant_x_ddd_2d646 : Constant  Value=x_ddd
  Constant_x_ddd_97782 : Constant  Value=x_ddd
  Constant_x_l_04055 : Constant  Value=x_l
  Constant_x_l_4c5bf : Constant  Value=x_l
  Constant_x_l_72b5b : Constant  Value=x_l
  Constant_x_l_772f0 : Constant  Value=x_l
  Constant_x_l_b1e67 : Constant  Value=x_l
  Constant_x_l_f7371 : Constant  Value=x_l
  Constant_x_qd_b23dd : Constant  Value=x_qd
  Constant_x_qd_b2dd2 : Constant  Value=x_qd
  Constant_x_qd_ecb1b : Constant  Value=x_qd
  Constant_x_qdd_05e86 : Constant  Value=x_qdd
  Constant_x_qdd_8a48b : Constant  Value=x_qdd
  Constant_x_qdd_92e19 : Constant  Value=x_qdd
  Divide_2d6e3 : Product  Inputs=*/
  Divide_34b98 : Product  Inputs=*/
  Divide_5c167 : Product  Inputs=*/
  Divide_5e907 : Product  Inputs=*/
  Divide_5f281 : Product  Inputs=*/
  Divide_864c0 : Product  Inputs=*/
  Divide_94b97 : Product  Inputs=*/
  Divide_b87e3 : Product  Inputs=*/
  Divide_c97bf : Product  Inputs=*/
  Divide_e48b5 : Product  Inputs=*/
  MathFunc_sqrt_41969 : Sqrt
  Power_0f973 : Math  Operator=pow
  Power_1ee58 : Math  Operator=pow
  Product_00f4a : Product
  Product_083ab : Product
  Product_13b78 : Product
  Product_1a6a8 : Product
  Product_1a877 : Product
  Product_1f579 : Product
  Product_308ee : Product
  Product_3c714 : Product
  Product_5f770 : Product
  Product_63fae : Product
  Product_6dc99 : Product
  Product_702db : Product
  Product_92ef1 : Product
  Product_9975e : Product
  Product_b8641 : Product
  Product_bb9b5 : Product
  Product_c42a4 : Product
  Product_cfe22 : Product
  Product_d9137 : Product
  Product_e4b2e : Product
  Product_e88df : Product
  Product_fd5e9 : Product
  Product_fea61 : Product
  Subtract_14511 : Sum  Inputs=+-
  Subtract_27d5c : Sum  Inputs=+-
  Subtract_7d8ca : Sum  Inputs=+-
  Subtract_9e610 : Sum  Inputs=+-
  Subtract_badd5 : Sum  Inputs=+-
  Subtract_c0f00 : Sum  Inputs=+-
  Subtract_c6082 : Sum  Inputs=+-
  Subtract_d72a4 : Sum  Inputs=+-
  Subtract_f7f6c : Sum  Inputs=+-
  Blockout_d_V_f_SG_D_2_347d2 : Outport
  wires:
  Constant_-1_8f530/1 -> Product_e88df/1
  Constant_2.0_35285/1 -> Product_5f770/1
  Constant_-1_3697e/1 -> Product_fd5e9/1
  Product_5f770/1 -> Product_1f579/1
  Product_fd5e9/1 -> Add_42a19/1
  Constant_x_l_f7371/1 -> Product_308ee/2
  Constant_x_l_04055/1 -> Product_fd5e9/2
  State_psi_1d_SG_D_2_f4f15/1 -> Product_e88df/2
  Constant_x_l_772f0/1 -> Subtract_c6082/2
  Constant_x_dd_29afe/1 -> Subtract_badd5/1
  Product_00f4a/1 -> Divide_5f281/1
  Constant_x_ddd_2d646/1 -> Subtract_badd5/2
  Constant_x_qd_b23dd/1 -> Add_f8b00/2
  Add_42a19/1 -> Product_cfe22/2
  Constant_x_qdd_92e19/1 -> Add_42a19/2
  Constant_-1_61211/1 -> Product_9975e/1
  Constant_x_dd_5f5ab/1 -> Subtract_c6082/1
  Subtract_27d5c/1 -> Add_f52c1/1
  Power_1ee58/1 -> Add_8b73e/1
  Constant_x_l_b1e67/1 -> Product_9975e/2
  Constant_2.0_28a57/1 -> Product_fea61/1
  Constant_x_qd_ecb1b/1 -> Subtract_f7f6c/1
  Constant_pi_76282/1 -> Product_fea61/2
  Subtract_9e610/1 -> Product_b8641/2
  Constant_x_qdd_05e86/1 -> Subtract_f7f6c/2
  State_psi_fd_SG_D_2_7e9d1/1 -> Product_bb9b5/1
  Constant_-1_fe762/1 -> Product_308ee/1
  Product_e88df/1 -> Product_e4b2e/1
  State_w_SG_D_2_2be4f/1 -> Product_083ab/2
  Subtract_badd5/1 -> Product_e4b2e/2
  Constant_x_dd_d62bf/1 -> Subtract_d72a4/1
  State_psi_q_SG_D_2_14f0d/1 -> Add_f52c1/2
  State_w_SG_D_2_bb1ed/1 -> Product_13b78/2
  Subtract_14511/1 -> Product_bb9b5/2
  Constant_x_l_4c5bf/1 -> Subtract_d72a4/2
  Add_6c81e/1 -> Add_215c6/1
  Constant_x_ddd_24596/1 -> Subtract_14511/1
  Constant_x_l_72b5b/1 -> Subtract_14511/2
  State_psi_gq_SG_D_2_56303/1 -> Product_cfe22/1
  Product_9975e/1 -> Add_f8a87/1
  Subtract_c6082/1 -> Divide_b87e3/2
  Constant_x_qd_b2dd2/1 -> Add_f8a87/2
  Product_13b78/1 -> Divide_c97bf/1
  State_psi_kq_SG_D_2_82247/1 -> Product_c42a4/1
  Subtract_f7f6c/1 -> Product_c42a4/2
  Product_bb9b5/1 -> Divide_b87e3/1
  State_V_f_SG_D_2_eb789/1 -> Subtract_7d8ca/2
  Product_308ee/1 -> Add_f8b00/1
  Product_e4b2e/1 -> Divide_5c167/1
  Divide_5e907/1 -> Subtract_27d5c/1
  Subtract_d72a4/1 -> Divide_5c167/2
  Product_cfe22/1 -> Divide_5e907/1
  Add_f8a87/1 -> Divide_5e907/2
  Product_c42a4/1 -> Divide_34b98/1
  Divide_b87e3/1 -> Subtract_9e610/2
  Constant_f0_e8267/1 -> Product_1f579/2
  Add_f8b00/1 -> Divide_34b98/2
  Divide_5c167/1 -> Add_eda87/1
  State_psi_d_SG_D_2_39d83/1 -> Add_eda87/2
  Divide_34b98/1 -> Subtract_27d5c/2
  Constant_-1_43789/1 -> Product_702db/1
  Constant_R_a_6bfc8/1 -> Product_702db/2
  Constant_f0_b4d8f/1 -> Product_3c714/2
  Add_eda87/1 -> Subtract_9e610/1
  Product_702db/1 -> Product_b8641/1
  Constant_pi_b9b82/1 -> Product_5f770/2
  State_psi_q_SG_D_2_09452/1 -> Product_13b78/1
  Constant_R_a_8a759/1 -> Product_00f4a/1
  State_E_fd_SG_D_2_4dd56/1 -> Product_63fae/2
  Add_f52c1/1 -> Product_00f4a/2
  State_psi_d_SG_D_2_84408/1 -> Product_083ab/1
  Product_fea61/1 -> Product_3c714/1
  Product_b8641/1 -> Divide_2d6e3/1
  Constant_x_ddd_97782/1 -> Divide_2d6e3/2
  Product_1f579/1 -> Divide_c97bf/2
  Constant_x_qdd_8a48b/1 -> Divide_5f281/2
  Product_083ab/1 -> Divide_94b97/1
  Product_3c714/1 -> Divide_94b97/2
  Divide_2d6e3/1 -> Add_86a6e/1
  Divide_c97bf/1 -> Add_86a6e/2
  Divide_5f281/1 -> Add_8eeac/1
  Divide_94b97/1 -> Add_8eeac/2
  Constant_-1_bf78f/1 -> Product_63fae/1
  Add_86a6e/1 -> Power_1ee58/1
  Constant_2.0_a953f/1 -> Power_1ee58/2
  Add_8eeac/1 -> Power_0f973/1
  Constant_2.0_e84b0/1 -> Power_0f973/2
  Product_63fae/1 -> Product_d9137/1
  Constant_K_A_8043f/1 -> Product_d9137/2
  Constant_K_s_edec8/1 -> Product_1a877/1
  State_Px_3_SG_D_2_3a9e9/1 -> Product_1a877/2
  Power_0f973/1 -> Add_8b73e/2
  Product_d9137/1 -> Product_6dc99/1
  Constant_K_F_9e071/1 -> Product_6dc99/2
  Product_1a877/1 -> Add_d67d9/1
  Constant_V_ref_66988/1 -> Add_d67d9/2
  Add_8b73e/1 -> MathFunc_sqrt_41969/1
  Product_6dc99/1 -> Divide_e48b5/1
  Constant_T_F_3c724/1 -> Divide_e48b5/2
  Constant_K_A_21356/1 -> Product_92ef1/1
  State_R_f_SG_D_2_e5370/1 -> Product_92ef1/2
  Add_d67d9/1 -> Subtract_c0f00/1
  MathFunc_sqrt_41969/1 -> Subtract_c0f00/2
  Divide_e48b5/1 -> Add_6c81e/1
  Product_92ef1/1 -> Add_6c81e/2
  Constant_K_A_28258/1 -> Product_1a6a8/1
  Subtract_c0f00/1 -> Product_1a6a8/2
  Product_1a6a8/1 -> Add_215c6/2
  Add_215c6/1 -> Subtract_7d8ca/1
  Subtract_7d8ca/1 -> Divide_864c0/1
  Constant_T_A_9adbf/1 -> Divide_864c0/2
  Divide_864c0/1 -> Blockout_d_V_f_SG_D_2_347d2/1

== system case1/SG_D_2/d_psi_1d_SG_D_2_block ==
  note: d_psi_1d_SG_D_2 in case1
      | $-\frac{\psi _{\mathrm{1d},\mathrm{SG},D,2}-\psi _{\mathrm{fd},\mathrm{SG},D,2}+\frac{\left(x_{\mathrm{dd}}-x_{l}\right)\,\left(\frac{\psi _{\mathrm{1d},\mathrm{SG},D,2}\,\left(x_{\mathrm{dd}}-x_{\mathrm{ddd}}\right)}{x_{\mathrm{dd}}-x_{l}}-\psi _{d,\mathrm{SG},D,2}+\frac{\psi _{\mathrm{fd},\mathrm{SG},D,2}\,\left(x_{\mathrm{ddd}}-x_{l}\right)}{x_{\mathrm{dd}}-x_{l}}\right)}{x_{\mathrm{ddd}}}}{T_{\mathrm{ddd}}}$
      | Automatically generated on 2025-10-31 18:48:22 .
  State_psi_1d_SG_D_2_96ec3 : Inport
  State_psi_fd_SG_D_2_d5601 : Inport  Port=2
  State_psi_1d_SG_D_2_3af5a : Inport  Port=3
  State_psi_d_SG_D_2_4d81a : Inport  Port=4
  State_psi_fd_SG_D_2_2bfe4 : Inport  Port=5
  Add_43765 : Sum
  Add_ddbef : Sum
  Add_f7acc : Sum
  Constant_-1_321f1 : Constant  Value=-1
  Constant_-1_60595 : Constant  Value=-1
  Constant_T_ddd_f64cb : Constant  Value=T_ddd
  Constant_x_dd_34b52 : Constant  Value=x_dd
  Constant_x_dd_5a898 : Constant  Value=x_dd
  Constant_x_dd_9b01a : Constant  Value=x_dd
  Constant_x_dd_e2350 : Constant  Value=x_dd
  Constant_x_ddd_143fa : Constant  Value=x_ddd
  Constant_x_ddd_4c3ae : Constant  Value=x_ddd
  Constant_x_ddd_d2f6a : Constant  Value=x_ddd
  Constant_x_l_6d1ba : Constant  Value=x_l
  Constant_x_l_6e452 : Constant  Value=x_l
  Constant_x_l_86593 : Constant  Value=x_l
  Constant_x_l_ef647 : Constant  Value=x_l
  Divide_17a30 : Product  Inputs=*/
  Divide_4754b : Product  Inputs=*/
  Divide_7ba5d : Product  Inputs=*/
  Divide_df273 : Product  Inputs=*/
  Product_2106f : Product
  Product_6a57d : Product
  Product_7d564 : Product
  Product_8848b : Product
  Product_dd9e6 : Product
  Subtract_22ca5 : Sum  Inputs=+-
  Subtract_40b7a : Sum  Inputs=+-
  Subtract_72954 : Sum  Inputs=+-
  Subtract_a953f : Sum  Inputs=+-
  Subtract_b5cb2 : Sum  Inputs=+-
  Subtract_fba9a : Sum  Inputs=+-
  Blockout_d_psi_1d_SG_D_2_57022 : Outport
  wires:
  Subtract_fba9a/1 -> Product_2106f/2
  Constant_x_l_ef647/1 -> Subtract_40b7a/2
  Divide_df273/1 -> Add_ddbef/2
  Subtract_a953f/1 -> Product_6a57d/2
  Constant_-1_60595/1 -> Product_dd9e6/1
  Constant_x_dd_e2350/1 -> Subtract_72954/1
  Divide_7ba5d/1 -> Blockout_d_psi_1d_SG_D_2_57022/1
  State_psi_fd_SG_D_2_d5601/1 -> Add_f7acc/2
  State_psi_1d_SG_D_2_3af5a/1 -> Product_dd9e6/2
  Divide_17a30/1 -> Subtract_a953f/2
  Constant_x_ddd_143fa/1 -> Subtract_72954/2
  State_psi_1d_SG_D_2_96ec3/1 -> Product_8848b/2
  Product_dd9e6/1 -> Product_7d564/1
  Subtract_72954/1 -> Product_7d564/2
  Constant_x_dd_5a898/1 -> Subtract_40b7a/1
  Constant_x_ddd_4c3ae/1 -> Subtract_fba9a/1
  Constant_x_l_86593/1 -> Subtract_fba9a/2
  Product_7d564/1 -> Divide_4754b/1
  Subtract_40b7a/1 -> Divide_4754b/2
  State_psi_fd_SG_D_2_2bfe4/1 -> Product_2106f/1
  Constant_x_dd_9b01a/1 -> Subtract_b5cb2/1
  Constant_x_l_6e452/1 -> Subtract_22ca5/2
  Constant_x_l_6d1ba/1 -> Subtract_b5cb2/2
  Constant_x_ddd_d2f6a/1 -> Divide_df273/2
  Divide_4754b/1 -> Add_43765/1
  State_psi_d_SG_D_2_4d81a/1 -> Add_43765/2
  Product_2106f/1 -> Divide_17a30/1
  Subtract_b5cb2/1 -> Divide_17a30/2
  Constant_x_dd_34b52/1 -> Subtract_22ca5/1
  Add_43765/1 -> Subtract_a953f/1
  Constant_-1_321f1/1 -> Product_8848b/1
  Subtract_22ca5/1 -> Product_6a57d/1
  Product_8848b/1 -> Add_f7acc/1
  Product_6a57d/1 -> Divide_df273/1
  Add_f7acc/1 -> Add_ddbef/1
  Add_ddbef/1 -> Divide_7ba5d/1
  Constant_T_ddd_f64cb/1 -> Divide_7ba5d/2
